simulink model "lab0_4"  (R2021a)
settings: Solver=VariableStepAuto  StartTime=0.0  StopTime=30.0  RelTol=1e-3
settings Model: Creator=Giancarlo  LastModifiedBy=Giancarlo

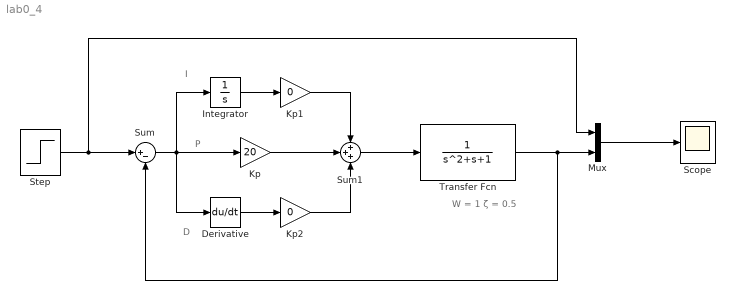
== system lab0_4 ==
  note: D
  note: P
  note: I
  note: W = 1
      | ζ = 0.5
  Derivative : Derivative
  Integrator : Integrator
  Kp : Gain  Gain=20
  Kp1 : Gain  Gain=0
  Kp2 : Gain  Gain=0
  Mux : Mux  Inputs=2
  Scope : Scope
  Step : Step  SampleTime=0
  Sum : Sum  Inputs=|+-
  Sum1 : Sum  Inputs=+++
  Transfer Fcn : TransferFcn  Denominator=[1 1 1]
  wires:
  Step/1 -> Mux/1, Sum/1
  Transfer Fcn/1 -> Sum/2, Mux/2
  Mux/1 -> Scope/1
  Sum/1 -> Derivative/1, Integrator/1, Kp/1
  Integrator/1 -> Kp1/1
  Sum1/1 -> Transfer Fcn/1
  Kp1/1 -> Sum1/1
  Kp/1 -> Sum1/2
  Kp2/1 -> Sum1/3
  Derivative/1 -> Kp2/1
